simulink model "mpcmonitorandtune"  (R2025a)
settings: Solver=FixedStepAuto  StartTime=0.0  StopTime=inf  FixedStep=0.02  RelTol=1e-3  EnableMultiTasking=on
InitFcn:
  | load2slx
model workspace (MAT data in the model file):
  F = [-0.8618  -0.0131  -0.1903; -0.0262  -0.9598  -0.0818; -0.139  0.0044  -0.6237; 0.76949416  0.02302564  0.28376223; 0.05909612  0.92119934  0.13451616; 0.20636922  -0.0051465  0.41509347; -0.703196288826  -0.030931828956  -0.325300738851; -0.093762205164  -0.8843494146  -0.17049782664; -0.235412147826  0.004062585186  -0.297744876105; 0.652041778329  0.0374689175646  0.339238548194; 0.127673420976  0.849276662584  0.196522224232; 0.244158287043  -0.00212544757986  0.23017009149; -0.610065448403  -0.0430117647626  -0.338731590381; -0.159596591925  -0.815943564776  -0.216337994265; -0.242353567764  -0.000145720570557  -0.189846546474]
  G = [1.8979  0.0281  -0.4399  0  0  0  0  0  0  0  0  0  0  0  0; -0.0159  -1.7644  -0.2623  0  0  0  0  0  0  0  0  0  0  0  0; 0.0655  0.0734  0.4799  0  0  0  0  0  0  0  0  0  0  0  0; -1.64786658  -0.01507096  0.29121698  1.8979  0.0281  -0.4399  0  0  0  0  0  0  0  0  0; -0.03982206  1.68673078  0.2240251  -0.0159  -1.7644  -0.2623  0  0  0  0  0  0  0  0  0; -0.30473041  -0.05744884  -0.23932165  0.0655  0.0734  0.4799  0  0  0  0  0  0  0  0  0; 1.47864328465  0.001824494362  -0.208362612179  -1.64786658  -0.01507096  0.29121698  1.8979  0.0281  -0.4399  0  0  0  0  0  0; 0.106322265122  -1.61383002838  -0.203072664886  -0.03982206  1.68673078  0.2240251  -0.0159  -1.7644  -0.2623  0  0  0  0  0  0; 0.418938594273  0.04534732038  0.109771463325  -0.30473041  -0.05744884  -0.23932165  0.0655  0.0734  0.4799  0  0  0  0  0  0; -1.35541161888  0.0109392290623  0.161337641615  1.47864328465  0.001824494362  -0.208362612179  -1.64786658  -0.01507096  0.29121698  1.8979  0.0281  -0.4399  0  0  0; -0.175057741134  1.54519684868  0.191388938497  0.106322265122  -1.61383002838  -0.203072664886  -0.03982206  1.68673078  0.2240251  -0.0159  -1.7644  -0.2623  0  0  0; -0.466355599848  -0.0356375805622  -0.0403955783084  0.418938594273  0.04534732038  0.109771463325  -0.30473041  -0.05744884  -0.23932165  0.0655  0.0734  0.4799  0  0  0; 1.25913446021  -0.0228876747426  -0.133860696086  -1.35541161888  0.0109392290623  0.161337641615  1.47864328465  0.001824494362  -0.208362612179  -1.64786658  -0.01507096  0.29121698  1.8979  0.0281  -0.4399; 0.241680092422  -1.48045138907  -0.184617791074  -0.175057741134  1.54519684868  0.191388938497  0.106322265122  -1.61383002838  -0.203072664886  -0.03982206  1.68673078  0.2240251  -0.0159  -1.7644  -0.2623; 0.478497948588  0.0275054722912  0.00361090133585  -0.466355599848  -0.0356375805622  -0.0403955783084  0.418938594273  0.04534732038  0.109771463325  -0.30473041  -0.05744884  -0.23932165  0.0655  0.0734  0.4799]
  H = [129.750680259 -7.60010398556 -19.5429084562 -100.35260221 7.92753113853 14.4815749694 74.3205001843 -7.58160232914 -10.6139187187 -49.5448089621 6.25955402468 7.17559354227 ... (225 elements, 15x15)]
  Pc = [-1.8979 0.0159 -0.0655 1.8979 -0.0159 0.0655 1.64786658 0.03982206 0.30473041 -1.64786658 -0.03982206 -0.30473041 ... (990 elements, 66x15)]
  Qvec = [10  0  0  0  0  0  0  0  0  0  0  0  0  0  0; 0  10  0  0  0  0  0  0  0  0  0  0  0  0  0; 0  0  10  0  0  0  0  0  0  0  0  0  0  0  0; 0  0  0  10  0  0  0  0  0  0  0  0  0  0  0; 0  0  0  0  10  0  0  0  0  0  0  0  0  0  0; 0  0  0  0  0  10  0  0  0  0  0  0  0  0  0; 0  0  0  0  0  0  10  0  0  0  0  0  0  0  0; 0  0  0  0  0  0  0  10  0  0  0  0  0  0  0; 0  0  0  0  0  0  0  0  10  0  0  0  0  0  0; 0  0  0  0  0  0  0  0  0  10  0  0  0  0  0; 0  0  0  0  0  0  0  0  0  0  10  0  0  0  0; 0  0  0  0  0  0  0  0  0  0  0  10  0  0  0; 0  0  0  0  0  0  0  0  0  0  0  0  10.2743328496  0.0454268079921  0.373732188276; 0  0  0  0  0  0  0  0  0  0  0  0  0.0454268079921  10.2974447606  0.1714057017; 0  0  0  0  0  0  0  0  0  0  0  0  0.373732188276  0.1714057017  11.3248324187]
  Sc = [-0.8618  -0.0131  -0.1903; -0.0262  -0.9598  -0.0818; -0.139  0.0044  -0.6237; 0.8618  0.0131  0.1903; 0.0262  0.9598  0.0818; 0.139  -0.0044  0.6237; 0.76949416  0.02302564  0.28376223; 0.05909612  0.92119934  0.13451616; 0.20636922  -0.0051465  0.41509347; -0.76949416  -0.02302564  -0.28376223; -0.05909612  -0.92119934  -0.13451616; -0.20636922  0.0051465  -0.41509347; -0.703196288826  -0.030931828956  -0.325300738851; -0.093762205164  -0.8843494146  -0.17049782664; -0.235412147826  0.004062585186  -0.297744876105; 0.703196288826  0.030931828956  0.325300738851; 0.093762205164  0.8843494146  0.17049782664; 0.235412147826  -0.004062585186  0.297744876105; 0.652041778329  0.0374689175646  0.339238548194; 0.127673420976  0.849276662584  0.196522224232; 0.244158287043  -0.00212544757986  0.23017009149; -0.652041778329  -0.0374689175646  -0.339238548194; -0.127673420976  -0.849276662584  -0.196522224232; -0.244158287043  0.00212544757986  -0.23017009149; -0.610065448403  -0.0430117647626  -0.338731590381; -0.159596591925  -0.815943564776  -0.216337994265; -0.242353567764  -0.000145720570557  -0.189846546474; 0.610065448403  0.0430117647626  0.338731590381; 0.159596591925  0.815943564776  0.216337994265; 0.242353567764  0.000145720570557  0.189846546474; 0  0  0; 0  0  0; 0  0  0; 0  0  0; 0  0  0; 0  0  0; 0  0  0; 0  0  0; 0  0  0; 0  0  0; 0  0  0; 0  0  0; 0  0  0; 0  0  0; 0  0  0; 0  0  0; 0  0  0; 0  0  0; 0  0  0; 0  0  0; 0  0  0; 0  0  0; 0  0  0; 0  0  0; 0  0  0; 0  0  0; 0  0  0; 0  0  0; 0  0  0; 0  0  0; -0.610065448403  -0.0430117647626  -0.338731590381; -0.159596591925  -0.815943564776  -0.216337994265; -0.242353567764  -0.000145720570557  -0.189846546474; 0.610065448403  0.0430117647626  0.338731590381; 0.159596591925  0.815943564776  0.216337994265; 0.242353567764  0.000145720570557  0.189846546474]
  m = 3
  nu = 15
  qc = [1; 1; 0.5; 1; 1; 0.5; 1; 1; 0.5; 1; 1; 0.5; 1; 1; 0.5; 1; 1; 0.5; 1; 1; 0.5; 1; 1; 0.5; 1; 1; 0.5; 1; 1; 0.5; 1.41421356237; 1.41421356237; 2; 1.41421356237; 1.41421356237; 2; 1.41421356237; 1.41421356237; 2; 1.41421356237; 1.41421356237; 2; 1.41421356237; 1.41421356237; 2; 1.41421356237; 1.41421356237; 2; 1.41421356237; 1.41421356237; 2; 1.41421356237; 1.41421356237; 2; 1.41421356237; 1.41421356237; 2; 1.41421356237; 1.41421356237; 2; 1; 1; 0.5; 1; 1; 0.5]
undefined symbols (not defined in the file or in its folder): dspblkCoreblockFVToolHelper, gcbh
libraries: px4Peripheralslib x1, px4Sensorslib x1
settings Model: SimulationMode=external  ExtModeTrigDuration=10  Creator=The MathWorks, Inc.  LastModifiedBy=aero
settings SolverCC: AlgebraicLoopSolver=TrustRegion  PositivePriorityOrder=on  AutoInsertRateTranBlk=on  MaxZcPerStep=1.0
settings OptimizationCC: EnhancedBackFolding=on  PassReuseOutputArgsAs=Individual arguments  MaxStackSize=64  OptimizeBlockOrder=speed  DifferentSizesBufferReuse=on  OptimizationCustomize=off  EfficientTunableParamExpr=on
settings DebuggingCC: ParameterPrecisionLossMsg=none  ParameterTunabilityLossMsg=error  UnconnectedInputMsg=warning  UnconnectedOutputMsg=warning  UnconnectedLineMsg=warning  SubsystemReferenceDiagnosticForUnitTest=warning  ArithmeticOperatorsInVariantConditions=warning
settings HardwareCC: ProdBitPerPointer=32.0  ProdBitPerSizeT=32.0  ProdBitPerPtrDiffT=32.0  ProdLargestAtomicInteger=Long  ProdLargestAtomicFloat=Double  ProdWordSize=32.0  ProdLongLongMode=on  ProdHWDeviceType=ARM Compatible->ARM Cortex
settings ModelReferenceCC: EnableRefExpFcnMdlSchedulingChecks=on
settings SFSimCC: MATLABDynamicMemAlloc=off  SimTargetLang=C++  SimDLTargetLibrary=mkl-dnn
settings RTWCC: SystemTargetFile=ert.tlc  HardwareBoard=PX4 Pixhawk 6c  TLCOptions="-aInlineSetEventsForThisBaseRateFcn=TLC_FALSE -aSuppressMultiTaskScheduler=TLC_FALSE  -aRateBasedStepFcn=0"  TemplateMakefile=ert_default_tmf  GenerateReport=on  Toolchain=GNU Tools for PX4 Autopilots  BuildConfiguration=Faster Runs  IncludeHyperlinkInReport=on  LaunchReport=on  TargetLang=C++  GenerateTraceInfo=on  GenerateTraceReport=on  GenerateTraceReportSl=on  GenerateTraceReportSf=on  GenerateTraceReportEml=on  GPUComputeCapability=3.5  DLArmComputeVersion=19.05  Description=Embedded Coder
settings CodeAppCC: ForceParamTrailComments=on  IgnoreCustomStorageClasses=off  OperatorAnnotations=on  SimulinkDataObjDesc=on  SFDataObjDesc=on  InsertBlockDesc=on
settings ERTTargetCC: ExtModeTransport=3.0  ExtModeStaticAllocSize=1024.0  InlinedParameterPlacement=Hierarchical

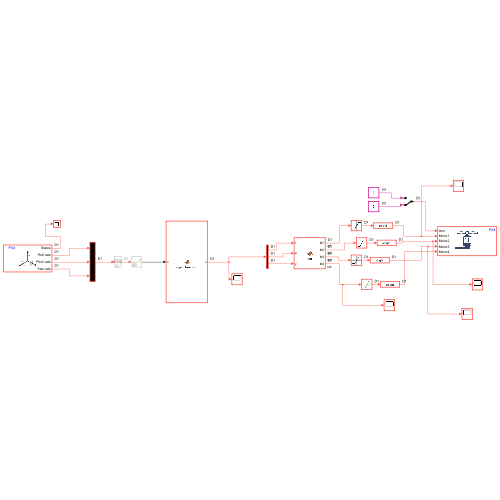
[thumbnail: Simulink's stored preview of the top-level diagram]
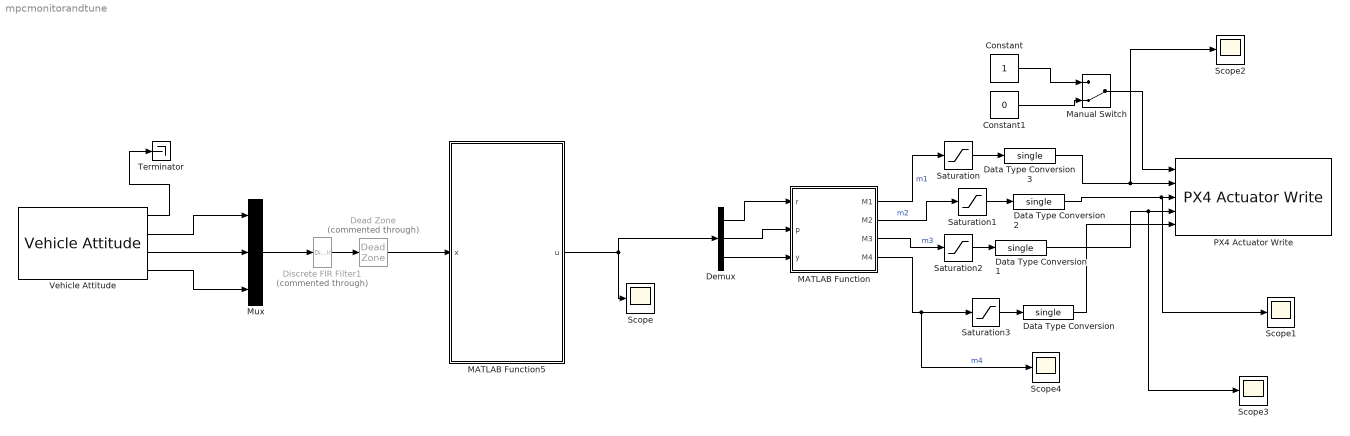
== system mpcmonitorandtune ==
  Constant : Constant  OutDataTypeStr=boolean
  Constant1 : Constant  Value=0  OutDataTypeStr=boolean
  Data Type Conversion{,1..3} (4 alike) : DataTypeConversion  OutDataTypeStr=single  SaturateOnIntegerOverflow=off  RndMeth=Floor
  Dead Zone : DeadZone  Commented=through  LowerValue=-0.017  UpperValue=0.017
  Demux : Demux  Outputs=3
  Discrete FIR Filter1 : DiscreteFir  Commented=through  LoadFcn=dspblkCoreblockFVToolHelper(gcbh,'load');  Coefficients=[0.2 0.2 0.2 0.2 0.2]
      settings: CopyFcn=dspblkCoreblockFVToolHelper(gcbh,'copy');  DeleteFcn=dspblkCoreblockFVToolHelper(gcbh,'close');  ModelCloseFcn=dspblkCoreblockFVToolHelper(gcbh,'close');  PreSaveFcn=dspblkCoreblockFVToolHelper(gcbh,'presave');  PostSaveFcn=dspblkCoreblockFVToolHelper(gcbh,'postsave');  CloseFcn=dspblkCoreblockFVToolHelper(gcbh,'close');
  MATLAB Function : MATLAB Function  TreatAsAtomicUnit=on  SystemSampleTime=0.02
  MATLAB Function5 : MATLAB Function  TreatAsAtomicUnit=on  SystemSampleTime=0.02
  Manual Switch : ManualSwitch  CurrentSetting=0
  Mux : Mux  Inputs=3
  PX4 Actuator Write : px4Peripheralslib/PX4 Actuator Write  Motor1Enable=on  Motor2Enable=on  Motor3Enable=on  Motor4Enable=on  Motor5Enable=off  Motor6Enable=off  Motor7Enable=off  Motor8Enable=off  Motor9Enable=off  Motor10Enable=off  Motor11Enable=off  Motor12Enable=off  IsMotorArray=off  Servo1Enable=off  Servo2Enable=off  Servo3Enable=off  Servo4Enable=off  Servo5Enable=off  Servo6Enable=off  Servo7Enable=off  Servo8Enable=off  IsServoArray=off
  Saturation{,1..3} (4 alike) : Saturate  UpperLimit=1  LowerLimit=0
  Scope{,1..4} (5 alike) : Scope
      Scope settings: ActiveDisplayYMinimum=-0.20094468799626919  ActiveDisplayYMaximum=0.25880684258194991
      Scope1 settings: ActiveDisplayYMinimum=0.20660063251852989  ActiveDisplayYMaximum=0.20984167233109474
      Scope2 settings: ActiveDisplayYMinimum=0.00829335488379003  ActiveDisplayYMaximum=0.64960764907300472  DataLoggingVariableName=ScopeData2
      Scope3 settings: ActiveDisplayYMinimum=0.086084697037949576  ActiveDisplayYMaximum=0.57265901246140893  DataLoggingVariableName=ScopeData3
      Scope4 settings: ActiveDisplayYMinimum=0.09643536073618425  ActiveDisplayYMaximum=0.86308686784221988  DataLoggingVariableName=ScopeData4
  Terminator : Terminator
  Vehicle Attitude : px4Sensorslib/Vehicle Attitude  rollRate=on  pitchRate=on  yawRate=on  quaternion=off  uorbTimeStamp=off  BlockingMode=off  BlockTimeout=0.001  sampleTime=0.02
  wires:
  MATLAB Function/2(M2) -> Saturation1/1  "m2"
  Demux/3 -> MATLAB Function/3(y)
  Demux/1 -> MATLAB Function/1(r)
  MATLAB Function5/1(u) -> Demux/1, Scope/1
  MATLAB Function/1(M1) -> Saturation/1  "m1"
  MATLAB Function/4(M4) -> Scope4/1, Saturation3/1  "m4"
  Demux/2 -> MATLAB Function/2(p)
  MATLAB Function/3(M3) -> Saturation2/1  "m3"
  Vehicle Attitude/1 -> Terminator/1
  Vehicle Attitude/2 -> Mux/1
  Vehicle Attitude/3 -> Mux/2
  Vehicle Attitude/4 -> Mux/3
  Saturation/1 -> Data Type Conversion3/1
  Saturation1/1 -> Data Type Conversion2/1
  Saturation2/1 -> Data Type Conversion1/1
  Saturation3/1 -> Data Type Conversion/1
  Discrete FIR Filter1/1 -> Dead Zone/1
  Mux/1 -> Discrete FIR Filter1/1
  Dead Zone/1 -> MATLAB Function5/1(x)
  Data Type Conversion/1 -> PX4 Actuator Write/5
  Data Type Conversion1/1 -> Scope3/1, PX4 Actuator Write/4
  Data Type Conversion2/1 -> Scope1/1, PX4 Actuator Write/3
  Data Type Conversion3/1 -> Scope2/1, PX4 Actuator Write/2
  Constant1/1 -> Manual Switch/2
  Constant/1 -> Manual Switch/1
  Manual Switch/1 -> PX4 Actuator Write/1

== matlab function mpcmonitorandtune/MATLAB Function ==
  data: M1 output; r input; p input; y input; M2 output; M3 output; M4 output
function [M1,M2,M3,M4] = fcn( r, p, y)
% t: thrust
% r: roll
% p: pitch
% y: yaw
persistent trim mixer thrust
% M1 = t + r + p - y;
% M2 = t - r - p - y;
% M3 = t - r + p + y;
% M4 = t + r - p + y;
trim = [0.1344;0.2078;0.1551;0.2548];
thrust = 0;
u = [r;p;y; thrust];
mixer = [1 -1 -1 1;
        1 -1 1 -1;
        -1 -1 1 1
        1 1 1 1];
M = mixer\u;
M1= M(1,1)+trim(1,1);
M2= M(2,1)+trim(2,1);
M3= M(3,1)+trim(3,1);
M4= M(4,1)+trim(4,1);

== matlab function mpcmonitorandtune/MATLAB Function5 ==
  data: x input; u output size=[m 1]; H parameter double; F parameter double; Qvec parameter double; G parameter double; Pc parameter double; qc parameter double; Sc parameter double
function u = mpc_function(x, H, F, Qvec, G, Pc, qc, Sc)
persistent opts x0 u_prev 
if isempty(u_prev)
    u_prev = zeros(3,1,'double');
end

if isempty(x0)
    x0 = zeros(15,1,'double'); % Esto tiene que ser N*m porque u tiene m componentes y son N instantes de tiempo
end
% uvec = zeros(nu,1);
% if isempty(ubias)
%     ubias = zeros(3,1,'double');        % integrador de bias
% end
% if isempty(x_lp)
%     x_lp = zeros(3,1);
% end
% === Construcción del QP ===
f = (2*x'*F'*Qvec*G)';

% Resolver QP
if isempty(opts)
opts = optimoptions('quadprog', 'Algorithm','active-set','Display','off');
end
[uvec,a,b] = quadprog(2*H,f, Pc,qc + Sc*x,[],[],[],[],x0, opts);

% Acción de control 
u_mpc = zeros(3,1);
if  b > 0
    uvec = double(uvec);
    u_mpc(:) = uvec(1:3);
    u_prev = u_mpc;
    x0= uvec;
else
    u_mpc = u_prev;
end
% % integrador de bias
% % -------- Filtro lento (PROMEDIO de rates) --------
% % Esto decide QUÉ se integra
% x_lp = beta * x_lp + (1 - beta) * x;
% Ts= 0.02;
% 
% % Integración del error de velocidad
% ubias =  ubias + Ki * x *Ts;
% 
% % Anti-windup (OBLIGATORIO)
% ubias = min(max(ubias, -biasmax), biasmax);

% ================== ACCIÓN FINAL ==================
u = u_mpc ;

end
